simulink model "simul2v1"  (R2023b)
settings: Solver=ode4  StartTime=0.0  StopTime=600  FixedStep=0.0002  RelTol=1e-3
InitFcn:
  | init2
values from neighbouring files (symbols this model uses):
  eps_capteur = 0    [init2.m]
  K_s = 50e-3    (= 0.05)    [init2.m]
  tau_IEPE = 1 / (2 * pi * f_c_IEPE)    (= 0.318309886184)    [init2.m]
libraries: simulink x1
settings Model: Creator=xavie  LastModifiedBy=xavie
settings DataIOCC: ReturnWorkspaceOutputs=off

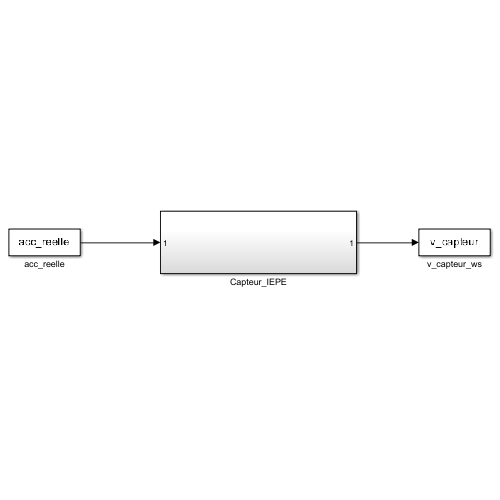
[thumbnail: Simulink's stored preview of the top-level diagram]
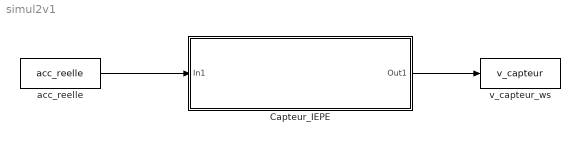
== system simul2v1 ==
  Capteur_IEPE : Subsystem
  acc_reelle : FromWorkspace  VariableName=acc_reelle  SampleTime=-1
  v_capteur_ws : ToWorkspace  VariableName=v_capteur  SampleTime=-1
  wires:
  acc_reelle/1 -> Capteur_IEPE/1(In1)
  Capteur_IEPE/1(Out1) -> v_capteur_ws/1

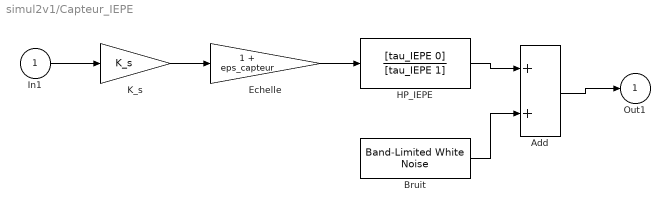
== system simul2v1/Capteur_IEPE ==
  In1 : Inport
  Add : Sum
  Bruit : simulink/Sources/Band-Limited White Noise  Cov=bruit_capteur_power  Ts=0.0002  seed=1234
  Echelle : Gain  Gain=1 + eps_capteur
  HP_IEPE : TransferFcn  Numerator=[tau_IEPE 0]  Denominator=[tau_IEPE 1]
  K_s : Gain  Gain=K_s
  Out1 : Outport
  wires:
  In1/1 -> K_s/1
  K_s/1 -> Echelle/1
  Echelle/1 -> HP_IEPE/1
  HP_IEPE/1 -> Add/1
  Bruit/1 -> Add/2
  Add/1 -> Out1/1
